simulink model "Area2"  (R2020a)
settings: Solver=VariableStepAuto  StartTime=0.0  StopTime=150  RelTol=1e-3
settings Model: Creator=prade  LastModifiedBy=prade

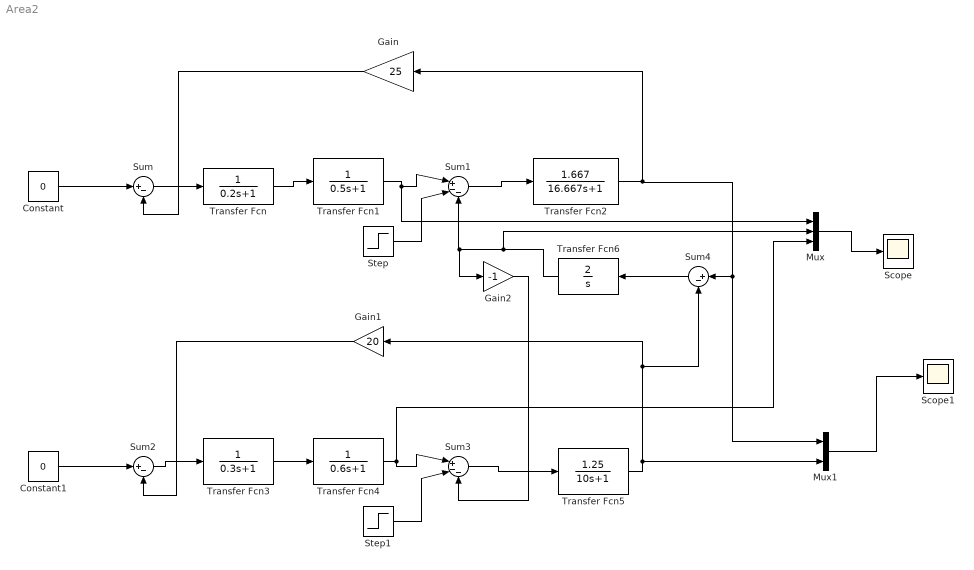
== system Area2 ==
  Constant : Constant  Value=0
  Constant1 : Constant  Value=0
  Gain : Gain  Gain=25
  Gain1 : Gain  Gain=20
  Gain2 : Gain  Gain=-1
  Mux : Mux  Inputs=3
  Mux1 : Mux  Inputs=2
  Scope : Scope
  Scope1 : Scope
  Step : Step  Before=0.2  After=0.2  SampleTime=0
  Step1 : Step  After=0  SampleTime=0
  Sum : Sum  Inputs=|+-
  Sum1 : Sum  Inputs=|+--
  Sum2 : Sum  Inputs=|+-
  Sum3 : Sum  Inputs=|+--
  Sum4 : Sum  Inputs=|+-
  Transfer Fcn : TransferFcn  Denominator=[0.2 1]
  Transfer Fcn1 : TransferFcn  Denominator=[0.5 1]
  Transfer Fcn2 : TransferFcn  Numerator=[1.667]  Denominator=[ 16.667 1]
  Transfer Fcn3 : TransferFcn  Denominator=[0.3 1]
  Transfer Fcn4 : TransferFcn  Denominator=[0.6 1]
  Transfer Fcn5 : TransferFcn  Numerator=[1.25]  Denominator=[10 1]
  Transfer Fcn6 : TransferFcn  Numerator=[2]  Denominator=[1 0]
  wires:
  Constant/1 -> Sum/1
  Sum/1 -> Transfer Fcn/1
  Transfer Fcn/1 -> Transfer Fcn1/1
  Transfer Fcn1/1 -> Mux/1, Sum1/1
  Step/1 -> Sum1/2
  Sum1/1 -> Transfer Fcn2/1
  Transfer Fcn2/1 -> Mux1/1, Sum4/1, Gain/1
  Gain/1 -> Sum/2
  Gain1/1 -> Sum2/2
  Transfer Fcn5/1 -> Sum4/2, Gain1/1, Mux1/2
  Sum3/1 -> Transfer Fcn5/1
  Step1/1 -> Sum3/2
  Transfer Fcn4/1 -> Sum3/1, Mux/3
  Transfer Fcn3/1 -> Transfer Fcn4/1
  Sum2/1 -> Transfer Fcn3/1
  Constant1/1 -> Sum2/1
  Gain2/1 -> Sum3/3
  Transfer Fcn6/1 -> Mux/2, Sum1/3, Gain2/1
  Sum4/1 -> Transfer Fcn6/1
  Mux/1 -> Scope/1
  Mux1/1 -> Scope1/1
